simulink model "LQR_NL"  (R2019b)
settings: Solver=VariableStepAuto  StartTime=0.0  StopTime=100.0  RelTol=1e-3
values from neighbouring files (symbols this model uses):
  K = lqr(A,B,Q,R)    [LQR.m]
settings Model: Creator=kathp  LastModifiedBy=Nevil Patel
settings DataIOCC: ReturnWorkspaceOutputs=off
settings DebuggingCC: ArithmeticOperatorsInVariantConditions=warning
settings SFSimCC: SimUseLocalCustomCode=off  CustomCodeUndefinedFunction=UseInterfaceOnly
settings RTWCC: RTWUseLocalCustomCode=off

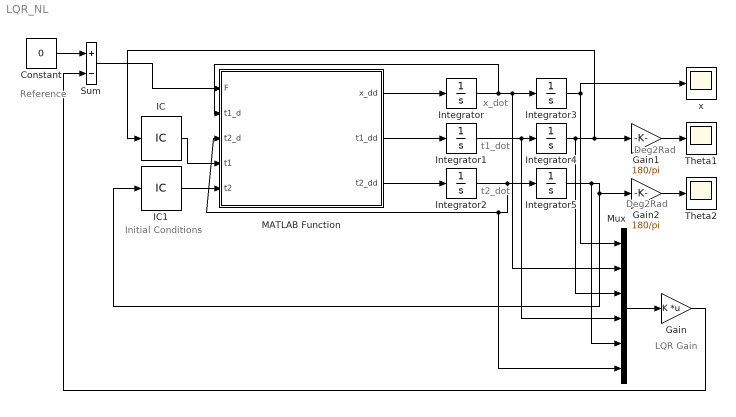
== system LQR_NL ==
  note: LQR Gain
  note: Deg2Rad
  note: t2_dot
  note: x_dot
  note: Reference
  note: Initial Conditions
  note: t1_dot
  note: Deg2Rad
  Constant : Constant  Value=0
  Gain : Gain  Gain=K  Multiplication=Matrix(K*u)
  Gain1 : Gain  Gain=180/pi
  Gain2 : Gain  Gain=180/pi
  IC : InitialCondition  Value=pi/10
  IC1 : InitialCondition  Value=pi/20
  Integrator{,1..5} (6 alike) : Integrator
  MATLAB Function : MATLAB Function  TreatAsAtomicUnit=on
  Mux : Mux  Inputs=6
  Sum : Sum  Inputs=|+-
  Theta1 : Scope
  Theta2 : Scope
  x : Scope
  wires:
  MATLAB Function/1(x_dd) -> Integrator/1
  MATLAB Function/2(t1_dd) -> Integrator1/1
  MATLAB Function/3(t2_dd) -> Integrator2/1
  Integrator/1 -> MATLAB Function/2(t1_d), Mux/2, Integrator3/1
  Integrator1/1 -> Mux/4, Integrator4/1
  Integrator2/1 -> MATLAB Function/3(t2_d), Mux/6, Integrator5/1
  Integrator3/1 -> Mux/1, x/1
  Integrator4/1 -> Mux/3, Gain1/1, IC/1
  Integrator5/1 -> Mux/5, IC1/1, Gain2/1
  Mux/1 -> Gain/1
  Constant/1 -> Sum/1
  Gain/1 -> Sum/2
  IC/1 -> MATLAB Function/4(t1)
  IC1/1 -> MATLAB Function/5(t2)
  Sum/1 -> MATLAB Function/1(F)
  Gain1/1 -> Theta1/1
  Gain2/1 -> Theta2/1

== matlab function LQR_NL/MATLAB Function ==
  data: F input; x_dd output; t1_d input; t2_d input; t1 input; t2 input; t1_dd output; t2_dd output
function [x_dd,t1_dd,t2_dd] = NonLinear_Estimation(F,t1_d,t2_d,t1,t2)

%% System Parameters
l1 = 20;
l2 = 10;
m1 = 100;
m2 = 100;
M = 1000;
g=9.8;

%% Variables
c1 = cos(t1);
c2 = cos(t2);
s1 = sin(t1);
s2 = sin(t2);

%% x_dd
x_dd = (F- (m1*l1*(t1_d^2)*(s1)) - (m2*l2*(t2_d^2)*(s2)) - m1*c1*s1*g - m2*c2*s2*g)/(M + m1*(s1^2) + m2*(s2^2));

%% t1_dd
t1_dd = (x_dd*c1 - g*s1)/l1;

%% t2_dd
t2_dd = (x_dd*c2 - g*s2)/l2;

end
